simulink model "ThermalModel"  (R2021a)
settings: Solver=FixedStepAuto  StartTime=0.0  StopTime=860  FixedStep=0.1  RelTol=1e-3
values from neighbouring files (symbols this model uses):
  ACderate = 0.7910    (= 0.791)    [simvar.m]
  airtemp = 20    [simvar.m]
  CoreDm = 0.07    [simvar.m]
  CoreRm = 0.250/2    (= 0.125)    [simvar.m]
  Di = 0.085    [Optomised_simvar.m]    (also in simvar.m)
  Dm = 0.08    [simvar.m]
  Hi = 0.250    (= 0.25)    [Optomised_simvar.m]    (also in simvar.m)
  La = 1    [Optomised_simvar.m]    (also in simvar.m = 1.5)
  Li = 0.488    [Optomised_simvar.m]    (also in simvar.m)
  Lw = 1    [Optomised_simvar.m]    (also in simvar.m = 1.5)
  Nl = 20    [simvar.m]
  Nt = 7    [simvar.m]
  Nv = 14    [simvar.m]
  PDi = 0.03    [Optomised_simvar.m]    (also in simvar.m = 0.01)
  PDm = 0.01    [simvar.m]
  PLi = 1    [Optomised_simvar.m]    (also in simvar.m = 3.2)
  PLm = 0.721    [simvar.m]
  PSplit = 0.95    [simvar.m]
  Rm = 0.268/2    (= 0.134)    [simvar.m]
  StartTempI = 295    [simvar.m]
  StartTempM = 291    [simvar.m]
libraries: fl_lib x50, nesl_utility x20
settings Model: Creator=Henry  LastModifiedBy=Henry
settings SolverCC: AlgebraicLoopSolver=TrustRegion
settings DataIOCC: ReturnWorkspaceOutputs=off
settings DebuggingCC: SFMachineParentedDataDiag=warning  ArithmeticOperatorsInVariantConditions=warning
settings SFSimCC: SimUseLocalCustomCode=off  CustomCodeUndefinedFunction=UseInterfaceOnly
settings RTWCC: RTWUseLocalCustomCode=off

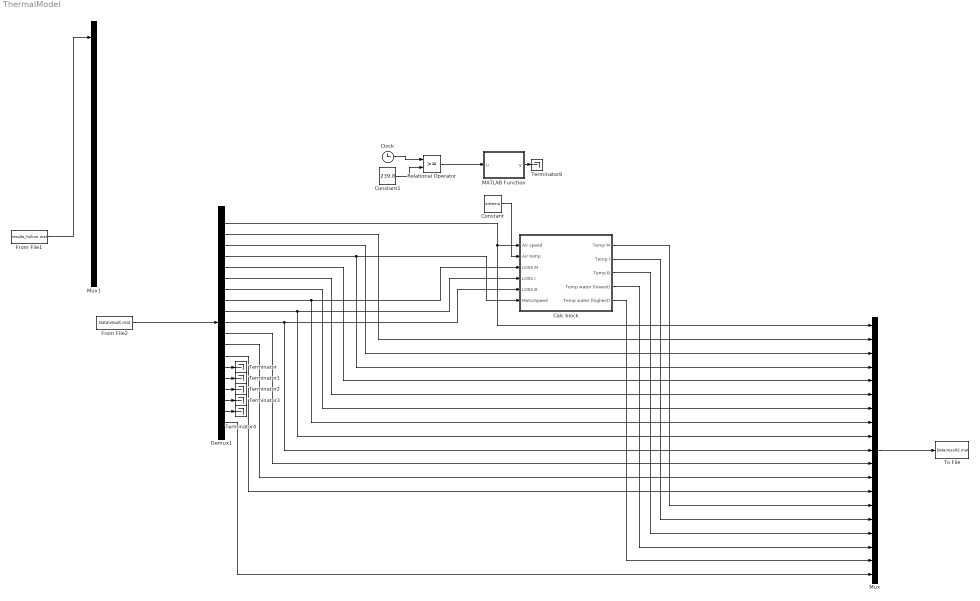
== system ThermalModel ==
  Calc block : Subsystem
  Clock : Clock
  Constant : Constant  Value=airtemp
  Constant1 : Constant  Value=239.8
  Demux1 : Demux  Outputs=19
  From File1 : FromFile  FileName=results_fullrun.mat  SampleTime=0
  From File2 : FromFile  FileName=Data\result.mat  SampleTime=0
  MATLAB Function : MATLAB Function  TreatAsAtomicUnit=on
  Mux : Mux  Inputs=19
  Mux1 : Mux  Inputs=8
  Relational Operator : RelationalOperator  OutDataTypeStr=boolean  RndMeth=Simplest
  Terminator{,1..4,8} (6 alike) : Terminator
  To File : ToFile  Filename=Data/result2.mat  MatrixName=Result  SaveFormat=Timeseries
  wires:
  Constant/1 -> Calc block/2(Air temp)
  Demux1/9 -> Calc block/4(LOSS I), Mux/9
  Demux1/8 -> Calc block/3(LOSS M), Mux/8
  Demux1/4 -> Calc block/6(MotorSpeed), Mux/4
  Demux1/10 -> Calc block/5(LOSS B), Mux/10
  Calc block/1(Temp M) -> Mux/14
  Calc block/2(Temp I) -> Mux/15
  Calc block/3(Temp B) -> Mux/16
  Calc block/4(Temp water (lowest)) -> Mux/17
  Calc block/5(Temp water (highest)) -> Mux/18
  Demux1/1 -> Mux/1, Calc block/1(Air speed)
  Clock/1 -> Relational Operator/1
  Constant1/1 -> Relational Operator/2
  Relational Operator/1 -> MATLAB Function/1(u)
  MATLAB Function/1(y) -> Terminator8/1
  Demux1/2 -> Mux/2
  Demux1/3 -> Mux/3
  Demux1/5 -> Mux/5
  Demux1/6 -> Mux/6
  Demux1/11 -> Mux/11
  Demux1/12 -> Mux/12
  Demux1/13 -> Mux/13
  Demux1/19 -> Mux/19
  Demux1/7 -> Mux/7
  Mux/1 -> To File/1
  Demux1/14 -> Terminator/1
  Demux1/15 -> Terminator1/1
  Demux1/16 -> Terminator2/1
  Demux1/17 -> Terminator3/1
  Demux1/18 -> Terminator4/1
  From File1/1 -> Mux1/1
  From File2/1 -> Demux1/1

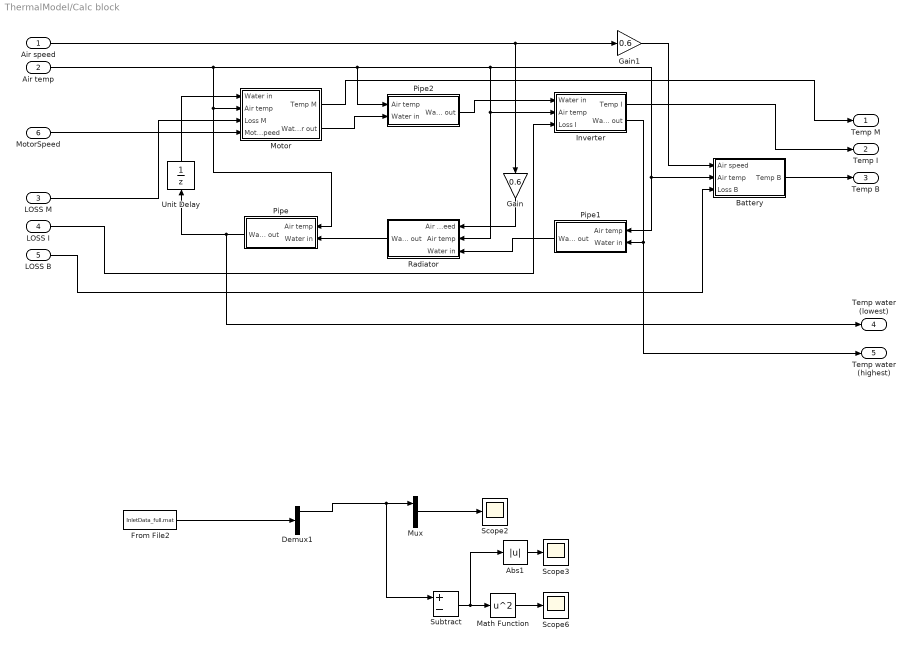
== system ThermalModel/Calc block ==
  Air speed : Inport
  Air temp : Inport  Port=2
  LOSS M : Inport  Port=3
  LOSS I : Inport  Port=4
  LOSS B : Inport  Port=5
  MotorSpeed : Inport  Port=6
  Abs1 : Abs
  Battery : Subsystem
  Demux1 : Demux  Outputs=3
  From File2 : FromFile  FileName=InletData_full.mat  SampleTime=0
  Gain : Gain  Gain=0.6
  Gain1 : Gain  Gain=0.6
  Inverter : Subsystem
  Math Function : Math  Operator=square  SaturateOnIntegerOverflow=on
  Motor : Subsystem
  Mux : Mux  Inputs=2
  Pipe : Subsystem
  Pipe1 : Subsystem
  Pipe2 : Subsystem
  Radiator : Subsystem
  Scope2 : Scope
  Scope3 : Scope
  Scope6 : Scope
  Subtract : Sum  Inputs=+-
  Unit Delay : UnitDelay  InitialCondition=20  SampleTime=-1  HasFrameUpgradeWarning=on
  Temp M : Outport  VectorParamsAs1DForOutWhenUnconnected=off
  Temp I : Outport  Port=2  VectorParamsAs1DForOutWhenUnconnected=off
  Temp B : Outport  Port=3  VectorParamsAs1DForOutWhenUnconnected=off
  Temp water (lowest) : Outport  Port=4  VectorParamsAs1DForOutWhenUnconnected=off
  Temp water (highest) : Outport  Port=5  VectorParamsAs1DForOutWhenUnconnected=off
  wires:
  Pipe/1(Water out) -> Unit Delay/1, Temp water (lowest)/1
  Battery/1(Temp B) -> Temp B/1
  Motor/1(Temp M) -> Temp M/1
  LOSS M/1 -> Motor/3(Loss M)
  Inverter/1(Temp I) -> Temp I/1
  LOSS B/1 -> Battery/3(Loss B)
  LOSS I/1 -> Inverter/3(Loss I)
  Air speed/1 -> Gain/1, Gain1/1
  Air temp/1 -> Pipe2/1(Air temp), Pipe1/1(Air temp), Battery/2(Air temp), Inverter/2(Air temp), Radiator/2(Air temp), Pipe/1(Air temp), Motor/2(Air temp)
  Pipe2/1(Water out) -> Inverter/1(Water in)
  Inverter/2(Water out) -> Pipe1/2(Water in), Temp water (highest)/1
  Motor/2(Water out) -> Pipe2/2(Water in)
  MotorSpeed/1 -> Motor/4(MotorSpeed)
  Unit Delay/1 -> Motor/1(Water in)
  Gain/1 -> Radiator/1(Air speed)
  Radiator/1(Water out) -> Pipe/2(Water in)
  Gain1/1 -> Battery/1(Air speed)
  Pipe1/1(Water out) -> Radiator/3(Water in)
  From File2/1 -> Demux1/1
  Demux1/1 -> Subtract/1, Mux/1
  Mux/1 -> Scope2/1
  Subtract/1 -> Abs1/1, Math Function/1
  Math Function/1 -> Scope6/1
  Abs1/1 -> Scope3/1

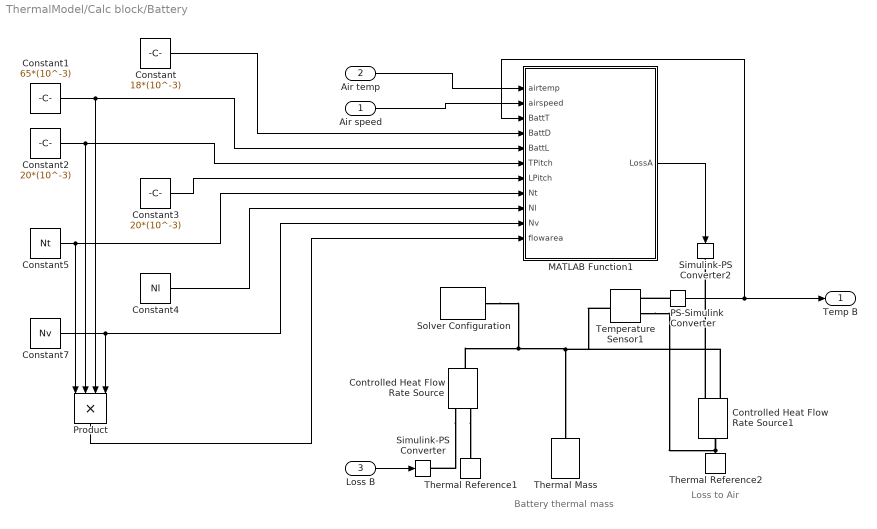
== system ThermalModel/Calc block/Battery ==
  note: Battery thermal mass
  note: Loss to Air
  Air speed : Inport
  Air temp : Inport  Port=2
  Loss B : Inport  Port=3
  Constant : Constant  Value=18*(10^-3)
  Constant1 : Constant  Value=65*(10^-3)
  Constant2 : Constant  Value=20*(10^-3)
  Constant3 : Constant  Value=20*(10^-3)
  Constant4 : Constant  Value=Nl
  Constant5 : Constant  Value=Nt
  Constant7 : Constant  Value=Nv
  Controlled Heat Flow Rate Source : fl_lib/Thermal/Thermal Sources/Controlled Heat Flow Rate Source
  Controlled Heat Flow Rate Source1 : fl_lib/Thermal/Thermal Sources/Controlled Heat Flow Rate Source
  MATLAB Function1 : MATLAB Function  TreatAsAtomicUnit=on
  PS-Simulink Converter : nesl_utility/PS-Simulink Converter  PhysicalDomain=network_engine_domain  SubClassName=ps_output  LeftPortType=input  RightPortType=output  PseudoPeriodic=off  Frequencies=[]  Unit=inherit  AffineConversion=off
      settings: SourceProductBaseCode=PW,SS
  Product : Product  Inputs=4
  Simulink-PS Converter : nesl_utility/Simulink-PS Converter  PhysicalDomain=network_engine_domain  SubClassName=ps_input  LeftPortType=input  RightPortType=output  PseudoPeriodic=off  Frequencies=[]  NoiseDistribution=none  NoiseParameters=[]  Unit=1  AffineConversion=off  FilteringAndDerivatives=provide  SimscapeFilterOrder=1  InputFilterTimeConstant=0.001  UdotUserProvided=0
      settings: SourceProductBaseCode=PW,SS
  Simulink-PS Converter2 : nesl_utility/Simulink-PS Converter  PhysicalDomain=network_engine_domain  SubClassName=ps_input  LeftPortType=input  RightPortType=output  PseudoPeriodic=off  Frequencies=[]  NoiseDistribution=none  NoiseParameters=[]  Unit=1  AffineConversion=off  FilteringAndDerivatives=provide  SimscapeFilterOrder=1  InputFilterTimeConstant=0.001  UdotUserProvided=0
      settings: SourceProductBaseCode=PW,SS
  Solver Configuration : nesl_utility/Solver Configuration  PhysicalDomain=network_engine_domain  SubClassName=solver  LeftPortType=input  RightPortType=generic  Tones=[]  Harmonics=[]  SimulateNoise=off  Profile=off  UseLocalSampling=off  EnableSwitchedLinearOptims=on  FrequencyDomain=off  UseCCode=off  RelTol=0.001  AbsTol=1e-06  MinStep=1e-09  ToWorkspace=off  RevertToSquareIcSolve=off  NumHomotopyIterations=100  PhasorMode=off  PhasorModeNumHarmonics=1  DoDC=off  ResidualTolerance=1e-09  UseLocalSolver=off  LocalSolverChoice=NE_BACKWARD_EULER_ADVANCER  LocalSolverSampleTime=0.001  DoFixedCost=off  MaxNonlinIter=3  MaxModeIter=2  ComputeImpulses=off  ImpulseIterations=2  LinearAlgebra=auto  EquationFormulation=NE_TIME_EF  DelaysMemoryBudget=2048  AutomaticFiltering=on  FilteringTimeConstant=0.001  PartitionStorageMethod=AS_NEEDED  PartitionMemoryBudget=1024  PartitionMethod=ROBUST
      settings: SourceProductBaseCode=PW,SS
  Temperature Sensor1 : fl_lib/Thermal/Thermal Sensors/Temperature Sensor
  Thermal Mass : fl_lib/Thermal/Thermal Elements/Thermal Mass  mass=Nt*Nl*Nv*0.045 kg  sp_heat=823 J/kg/K  T_specify=on  T_priority=High  T=300 K  T_nominal_specify=off  T_nominal_unit=K  T_nominal_value=1  Q_specify=off  Q_priority=None  Q=0 W  Q_nominal_specify=off  Q_nominal_unit=W  Q_nominal_value=1
  Thermal Reference1 : fl_lib/Thermal/Thermal Elements/Thermal Reference
  Thermal Reference2 : fl_lib/Thermal/Thermal Elements/Thermal Reference
  Temp B : Outport  VectorParamsAs1DForOutWhenUnconnected=off
  wires:
  Air temp/1 -> MATLAB Function1/1(airtemp)
  Air speed/1 -> MATLAB Function1/2(airspeed)
  Loss B/1 -> Simulink-PS Converter/1
  MATLAB Function1/1(LossA) -> Simulink-PS Converter2/1
  PS-Simulink Converter/1 -> Temp B/1, MATLAB Function1/3(BattT)
  Constant/1 -> MATLAB Function1/4(BattD)
  Constant1/1 -> MATLAB Function1/5(BattL), Product/3
  Constant2/1 -> MATLAB Function1/6(TPitch), Product/2
  Constant3/1 -> MATLAB Function1/7(LPitch)
  Constant5/1 -> MATLAB Function1/8(Nt), Product/1
  Constant4/1 -> MATLAB Function1/9(Nl)
  Product/1 -> MATLAB Function1/11(flowarea)
  Constant7/1 -> MATLAB Function1/10(Nv), Product/4
  connections:
  Controlled Heat Flow Rate Source/LConn1 -- Solver Configuration/RConn1 -- Temperature Sensor1/LConn1 -- Controlled Heat Flow Rate Source1/RConn2 -- Thermal Mass/LConn1
  Controlled Heat Flow Rate Source/RConn2 -- Thermal Reference1/LConn1
  Controlled Heat Flow Rate Source/RConn1 -- Simulink-PS Converter/RConn1
  Controlled Heat Flow Rate Source1/RConn1 -- Simulink-PS Converter2/RConn1
  Thermal Reference2/LConn1 -- Temperature Sensor1/RConn1 -- Controlled Heat Flow Rate Source1/LConn1
  PS-Simulink Converter/LConn1 -- Temperature Sensor1/RConn2

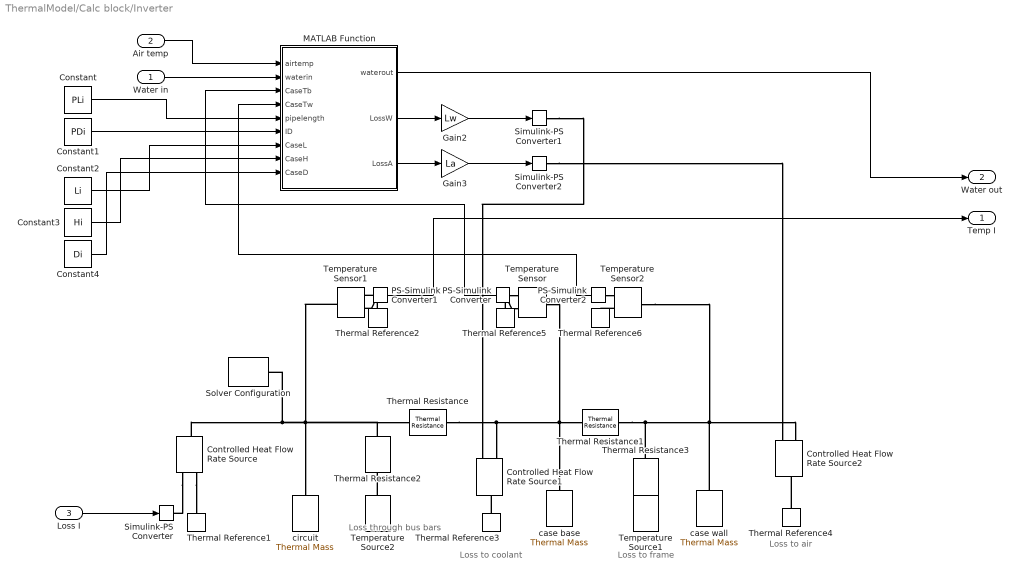
== system ThermalModel/Calc block/Inverter ==
  note: Loss to coolant
  note: Loss to air
  note: Loss through
      | bus bars
  note: Loss to frame
  Water in : Inport
  Air temp : Inport  Port=2
  Loss I : Inport  Port=3
  " case base" : fl_lib/Thermal/Thermal Elements/Thermal Mass  mass=MIbf kg  sp_heat=CpIb J/kg/K  T_specify=on  T_priority=High  T=StartTempI K  T_nominal_specify=off  T_nominal_unit=K  T_nominal_value=1  Q_specify=off  Q_priority=None  Q=0 W  Q_nominal_specify=off  Q_nominal_unit=W  Q_nominal_value=1
  " case wall" : fl_lib/Thermal/Thermal Elements/Thermal Mass  mass=MIbw kg  sp_heat=CpIb J/kg/K  T_specify=on  T_priority=High  T=StartTempI K  T_nominal_specify=off  T_nominal_unit=K  T_nominal_value=1  Q_specify=off  Q_priority=None  Q=0 W  Q_nominal_specify=off  Q_nominal_unit=W  Q_nominal_value=1
  Constant : Constant  Value=PLi
  Constant1 : Constant  Value=PDi
  Constant2 : Constant  Value=Li
  Constant3 : Constant  Value=Hi
  Constant4 : Constant  Value=Di
  Controlled Heat Flow Rate Source : fl_lib/Thermal/Thermal Sources/Controlled Heat Flow Rate Source
  Controlled Heat Flow Rate Source1 : fl_lib/Thermal/Thermal Sources/Controlled Heat Flow Rate Source
  Controlled Heat Flow Rate Source2 : fl_lib/Thermal/Thermal Sources/Controlled Heat Flow Rate Source
  Gain2 : Gain  Gain=Lw
  Gain3 : Gain  Gain=La
  MATLAB Function : MATLAB Function  TreatAsAtomicUnit=on
  PS-Simulink Converter : nesl_utility/PS-Simulink Converter  PhysicalDomain=network_engine_domain  SubClassName=ps_output  LeftPortType=input  RightPortType=output  PseudoPeriodic=off  Frequencies=[]  Unit=inherit  AffineConversion=off
      settings: SourceProductBaseCode=PW,SS
  PS-Simulink Converter1 : nesl_utility/PS-Simulink Converter  PhysicalDomain=network_engine_domain  SubClassName=ps_output  LeftPortType=input  RightPortType=output  PseudoPeriodic=off  Frequencies=[]  Unit=inherit  AffineConversion=off
      settings: SourceProductBaseCode=PW,SS
  PS-Simulink Converter2 : nesl_utility/PS-Simulink Converter  PhysicalDomain=network_engine_domain  SubClassName=ps_output  LeftPortType=input  RightPortType=output  PseudoPeriodic=off  Frequencies=[]  Unit=inherit  AffineConversion=off
      settings: SourceProductBaseCode=PW,SS
  Simulink-PS Converter : nesl_utility/Simulink-PS Converter  PhysicalDomain=network_engine_domain  SubClassName=ps_input  LeftPortType=input  RightPortType=output  PseudoPeriodic=off  Frequencies=[]  NoiseDistribution=none  NoiseParameters=[]  Unit=1  AffineConversion=off  FilteringAndDerivatives=provide  SimscapeFilterOrder=1  InputFilterTimeConstant=0.001  UdotUserProvided=0
      settings: SourceProductBaseCode=PW,SS
  Simulink-PS Converter1 : nesl_utility/Simulink-PS Converter  PhysicalDomain=network_engine_domain  SubClassName=ps_input  LeftPortType=input  RightPortType=output  PseudoPeriodic=off  Frequencies=[]  NoiseDistribution=none  NoiseParameters=[]  Unit=1  AffineConversion=off  FilteringAndDerivatives=provide  SimscapeFilterOrder=1  InputFilterTimeConstant=0.001  UdotUserProvided=0
      settings: SourceProductBaseCode=PW,SS
  Simulink-PS Converter2 : nesl_utility/Simulink-PS Converter  PhysicalDomain=network_engine_domain  SubClassName=ps_input  LeftPortType=input  RightPortType=output  PseudoPeriodic=off  Frequencies=[]  NoiseDistribution=none  NoiseParameters=[]  Unit=1  AffineConversion=off  FilteringAndDerivatives=provide  SimscapeFilterOrder=1  InputFilterTimeConstant=0.001  UdotUserProvided=0
      settings: SourceProductBaseCode=PW,SS
  Solver Configuration : nesl_utility/Solver Configuration  PhysicalDomain=network_engine_domain  SubClassName=solver  LeftPortType=input  RightPortType=generic  Tones=[]  Harmonics=[]  SimulateNoise=off  Profile=off  UseLocalSampling=off  EnableSwitchedLinearOptims=on  FrequencyDomain=off  UseCCode=off  RelTol=0.001  AbsTol=1e-06  MinStep=1e-09  ToWorkspace=off  RevertToSquareIcSolve=off  NumHomotopyIterations=100  PhasorMode=off  PhasorModeNumHarmonics=1  DoDC=off  ResidualTolerance=1e-09  UseLocalSolver=off  LocalSolverChoice=NE_BACKWARD_EULER_ADVANCER  LocalSolverSampleTime=0.001  DoFixedCost=off  MaxNonlinIter=3  MaxModeIter=2  ComputeImpulses=off  ImpulseIterations=2  LinearAlgebra=auto  EquationFormulation=NE_TIME_EF  DelaysMemoryBudget=2048  AutomaticFiltering=on  FilteringTimeConstant=0.001  PartitionStorageMethod=AS_NEEDED  PartitionMemoryBudget=1024  PartitionMethod=ROBUST
      settings: SourceProductBaseCode=PW,SS
  Temperature Sensor : fl_lib/Thermal/Thermal Sensors/Temperature Sensor
  Temperature Sensor1 : fl_lib/Thermal/Thermal Sensors/Temperature Sensor
  Temperature Sensor2 : fl_lib/Thermal/Thermal Sensors/Temperature Sensor
  Temperature Source1 : fl_lib/Thermal/Thermal Sources/Temperature Source  temperature=293.15 K
  Temperature Source2 : fl_lib/Thermal/Thermal Sources/Temperature Source  temperature=293.15 K
  Thermal Reference{1..6} (6 alike) : fl_lib/Thermal/Thermal Elements/Thermal Reference
  Thermal Resistance : fl_lib/Thermal/Thermal Elements/Thermal Resistance  resistance=Rcb K/W  T_specify=off  T_priority=None  T=0 K  T_nominal_specify=off  T_nominal_unit=K  T_nominal_value=1  Q_specify=off  Q_priority=None  Q=0 W  Q_nominal_specify=off  Q_nominal_unit=W  Q_nominal_value=1
      settings: SourceProductBaseCode=SS
  Thermal Resistance1 : fl_lib/Thermal/Thermal Elements/Thermal Resistance  resistance=Rba K/W  T_specify=off  T_priority=None  T=0 K  T_nominal_specify=off  T_nominal_unit=K  T_nominal_value=1  Q_specify=off  Q_priority=None  Q=0 W  Q_nominal_specify=off  Q_nominal_unit=W  Q_nominal_value=1
      settings: SourceProductBaseCode=SS
  Thermal Resistance2 : fl_lib/Thermal/Thermal Elements/Thermal Resistance  resistance=Rcbb K/W  T_specify=off  T_priority=None  T=0 K  T_nominal_specify=off  T_nominal_unit=K  T_nominal_value=1  Q_specify=off  Q_priority=None  Q=0 W  Q_nominal_specify=off  Q_nominal_unit=W  Q_nominal_value=1
      settings: SourceProductBaseCode=SS
  Thermal Resistance3 : fl_lib/Thermal/Thermal Elements/Thermal Resistance  resistance=Rcf K/W  T_specify=off  T_priority=None  T=0 K  T_nominal_specify=off  T_nominal_unit=K  T_nominal_value=1  Q_specify=off  Q_priority=None  Q=0 W  Q_nominal_specify=off  Q_nominal_unit=W  Q_nominal_value=1
      settings: SourceProductBaseCode=SS
  circuit : fl_lib/Thermal/Thermal Elements/Thermal Mass  mass=MIc kg  sp_heat=CpIc J/kg/K  T_specify=on  T_priority=High  T=StartTempI K  T_nominal_specify=off  T_nominal_unit=K  T_nominal_value=1  Q_specify=off  Q_priority=None  Q=0 W  Q_nominal_specify=off  Q_nominal_unit=W  Q_nominal_value=1
  Temp I : Outport  VectorParamsAs1DForOutWhenUnconnected=off
  Water out : Outport  Port=2  VectorParamsAs1DForOutWhenUnconnected=off
  wires:
  PS-Simulink Converter1/1 -> Temp I/1
  Air temp/1 -> MATLAB Function/1(airtemp)
  Water in/1 -> MATLAB Function/2(waterin)
  MATLAB Function/1(waterout) -> Water out/1
  PS-Simulink Converter/1 -> MATLAB Function/3(CaseTb)
  MATLAB Function/2(LossW) -> Gain2/1
  MATLAB Function/3(LossA) -> Gain3/1
  Constant/1 -> MATLAB Function/5(pipelength)
  Constant1/1 -> MATLAB Function/6(ID)
  Constant2/1 -> MATLAB Function/7(CaseL)
  Constant3/1 -> MATLAB Function/8(CaseH)
  Constant4/1 -> MATLAB Function/9(CaseD)
  PS-Simulink Converter2/1 -> MATLAB Function/4(CaseTw)
  Loss I/1 -> Simulink-PS Converter/1
  Gain2/1 -> Simulink-PS Converter1/1
  Gain3/1 -> Simulink-PS Converter2/1
  connections:
  Thermal Reference3/LConn1 -- Controlled Heat Flow Rate Source1/LConn1
  Thermal Resistance/RConn1 -- Temperature Sensor/LConn1 -- Thermal Resistance1/LConn1 -- " case base"/LConn1 -- Controlled Heat Flow Rate Source1/RConn2
  PS-Simulink Converter/LConn1 -- Temperature Sensor/RConn2
  Controlled Heat Flow Rate Source/RConn2 -- Thermal Reference1/LConn1
  Controlled Heat Flow Rate Source/RConn1 -- Simulink-PS Converter/RConn1
  Thermal Resistance1/RConn1 -- Thermal Resistance3/LConn1 -- Temperature Sensor2/LConn1 -- " case wall"/LConn1 -- Controlled Heat Flow Rate Source2/RConn2
  PS-Simulink Converter1/LConn1 -- Temperature Sensor1/RConn2
  Simulink-PS Converter1/RConn1 -- Controlled Heat Flow Rate Source1/RConn1
  Simulink-PS Converter2/RConn1 -- Controlled Heat Flow Rate Source2/RConn1
  Thermal Reference4/LConn1 -- Controlled Heat Flow Rate Source2/LConn1
  Thermal Reference2/LConn1 -- Temperature Sensor1/RConn1
  Thermal Reference5/LConn1 -- Temperature Sensor/RConn1
  Controlled Heat Flow Rate Source/LConn1 -- Thermal Resistance2/LConn1 -- Thermal Resistance/LConn1 -- Temperature Sensor1/LConn1 -- circuit/LConn1 -- Solver Configuration/RConn1
  PS-Simulink Converter2/LConn1 -- Temperature Sensor2/RConn2
  Temperature Sensor2/RConn1 -- Thermal Reference6/LConn1
  Temperature Source1/LConn1 -- Thermal Resistance3/RConn1
  Temperature Source2/LConn1 -- Thermal Resistance2/RConn1

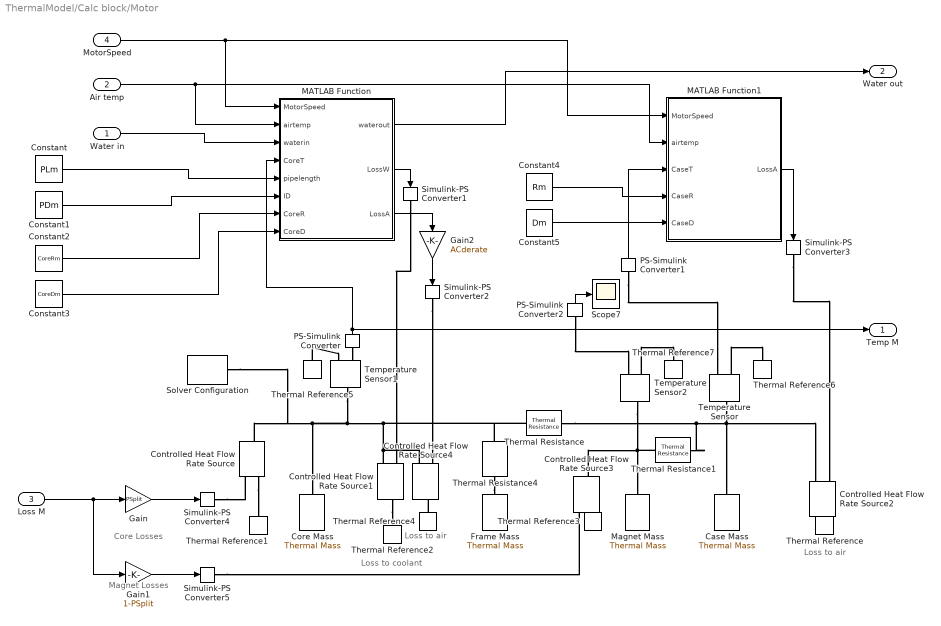
== system ThermalModel/Calc block/Motor ==
  note: Core Losses
  note: Loss to air
  note: Loss to coolant
  note: Loss to air
  note: Magnet Losses
  Water in : Inport
  Air temp : Inport  Port=2
  Loss M : Inport  Port=3
  MotorSpeed : Inport  Port=4
  " Case Mass" : fl_lib/Thermal/Thermal Elements/Thermal Mass  mass=Mcase kg  sp_heat=Cpcase J/kg/K  T_specify=on  T_priority=High  T=StartTempM K  T_nominal_specify=off  T_nominal_unit=K  T_nominal_value=1  Q_specify=off  Q_priority=None  Q=0 W  Q_nominal_specify=off  Q_nominal_unit=W  Q_nominal_value=1
  " Frame Mass" : fl_lib/Thermal/Thermal Elements/Thermal Mass  mass=30 kg  sp_heat=447 J/kg/K  T_specify=on  T_priority=High  T=StartTempM K  T_nominal_specify=off  T_nominal_unit=K  T_nominal_value=1  Q_specify=off  Q_priority=None  Q=0 W  Q_nominal_specify=off  Q_nominal_unit=W  Q_nominal_value=1
  " Magnet Mass" : fl_lib/Thermal/Thermal Elements/Thermal Mass  mass=Mmag kg  sp_heat=Cpmag J/kg/K  T_specify=on  T_priority=High  T=StartTempM K  T_nominal_specify=off  T_nominal_unit=K  T_nominal_value=1  Q_specify=off  Q_priority=None  Q=0 W  Q_nominal_specify=off  Q_nominal_unit=W  Q_nominal_value=1
  Constant : Constant  Value=PLm
  Constant1 : Constant  Value=PDm
  Constant2 : Constant  Value=CoreRm
  Constant3 : Constant  Value=CoreDm
  Constant4 : Constant  Value=Rm
  Constant5 : Constant  Value=Dm
  Controlled Heat Flow Rate Source{,1..4} (5 alike) : fl_lib/Thermal/Thermal Sources/Controlled Heat Flow Rate Source
  Core Mass : fl_lib/Thermal/Thermal Elements/Thermal Mass  mass=Mc kg  sp_heat=Cpcore J/kg/K  T_specify=on  T_priority=High  T=StartTempM K  T_nominal_specify=off  T_nominal_unit=K  T_nominal_value=1  Q_specify=off  Q_priority=None  Q=0 W  Q_nominal_specify=off  Q_nominal_unit=W  Q_nominal_value=1
  Gain : Gain  Gain=PSplit
  Gain1 : Gain  Gain=1-PSplit
  Gain2 : Gain  Gain=ACderate
  MATLAB Function : MATLAB Function  TreatAsAtomicUnit=on
  MATLAB Function1 : MATLAB Function  TreatAsAtomicUnit=on
  PS-Simulink Converter : nesl_utility/PS-Simulink Converter  PhysicalDomain=network_engine_domain  SubClassName=ps_output  LeftPortType=input  RightPortType=output  PseudoPeriodic=off  Frequencies=[]  Unit=inherit  AffineConversion=off
      settings: SourceProductBaseCode=PW,SS
  PS-Simulink Converter1 : nesl_utility/PS-Simulink Converter  PhysicalDomain=network_engine_domain  SubClassName=ps_output  LeftPortType=input  RightPortType=output  PseudoPeriodic=off  Frequencies=[]  Unit=inherit  AffineConversion=off
      settings: SourceProductBaseCode=PW,SS
  PS-Simulink Converter2 : nesl_utility/PS-Simulink Converter  PhysicalDomain=network_engine_domain  SubClassName=ps_output  LeftPortType=input  RightPortType=output  PseudoPeriodic=off  Frequencies=[]  Unit=inherit  AffineConversion=off
      settings: SourceProductBaseCode=PW,SS
  Scope7 : Scope
  Simulink-PS Converter{1..5} (5 alike) : nesl_utility/Simulink-PS Converter  PhysicalDomain=network_engine_domain  SubClassName=ps_input  LeftPortType=input  RightPortType=output  PseudoPeriodic=off  Frequencies=[]  NoiseDistribution=none  NoiseParameters=[]  Unit=1  AffineConversion=off  FilteringAndDerivatives=provide  SimscapeFilterOrder=1  InputFilterTimeConstant=0.001  UdotUserProvided=0
      settings: SourceProductBaseCode=PW,SS
  Solver Configuration : nesl_utility/Solver Configuration  PhysicalDomain=network_engine_domain  SubClassName=solver  LeftPortType=input  RightPortType=generic  Tones=[]  Harmonics=[]  SimulateNoise=off  Profile=off  UseLocalSampling=off  EnableSwitchedLinearOptims=on  FrequencyDomain=off  UseCCode=off  RelTol=0.001  AbsTol=1e-06  MinStep=1e-09  ToWorkspace=off  RevertToSquareIcSolve=off  NumHomotopyIterations=100  PhasorMode=off  PhasorModeNumHarmonics=1  DoDC=off  ResidualTolerance=1e-09  UseLocalSolver=off  LocalSolverChoice=NE_BACKWARD_EULER_ADVANCER  LocalSolverSampleTime=0.001  DoFixedCost=off  MaxNonlinIter=3  MaxModeIter=2  ComputeImpulses=off  ImpulseIterations=2  LinearAlgebra=auto  EquationFormulation=NE_TIME_EF  DelaysMemoryBudget=2048  AutomaticFiltering=on  FilteringTimeConstant=0.001  PartitionStorageMethod=AS_NEEDED  PartitionMemoryBudget=1024  PartitionMethod=ROBUST
      settings: SourceProductBaseCode=PW,SS
  Temperature Sensor : fl_lib/Thermal/Thermal Sensors/Temperature Sensor
  Temperature Sensor1 : fl_lib/Thermal/Thermal Sensors/Temperature Sensor
  Temperature Sensor2 : fl_lib/Thermal/Thermal Sensors/Temperature Sensor
  Thermal Reference{,1..7} (8 alike) : fl_lib/Thermal/Thermal Elements/Thermal Reference
  Thermal Resistance : fl_lib/Thermal/Thermal Elements/Thermal Resistance  resistance=Rcc K/W  T_specify=off  T_priority=None  T=0 K  T_nominal_specify=off  T_nominal_unit=K  T_nominal_value=1  Q_specify=off  Q_priority=None  Q=0 W  Q_nominal_specify=off  Q_nominal_unit=W  Q_nominal_value=1
      settings: SourceProductBaseCode=SS
  Thermal Resistance1 : fl_lib/Thermal/Thermal Elements/Thermal Resistance  resistance=Rmc K/W  T_specify=off  T_priority=None  T=0 K  T_nominal_specify=off  T_nominal_unit=K  T_nominal_value=1  Q_specify=off  Q_priority=None  Q=0 W  Q_nominal_specify=off  Q_nominal_unit=W  Q_nominal_value=1
      settings: SourceProductBaseCode=SS
  Thermal Resistance4 : fl_lib/Thermal/Thermal Elements/Thermal Resistance  resistance=Rcf K/W  T_specify=off  T_priority=None  T=0 K  T_nominal_specify=off  T_nominal_unit=K  T_nominal_value=1  Q_specify=off  Q_priority=None  Q=0 W  Q_nominal_specify=off  Q_nominal_unit=W  Q_nominal_value=1
      settings: SourceProductBaseCode=SS
  Temp M : Outport  VectorParamsAs1DForOutWhenUnconnected=off
  Water out : Outport  Port=2  VectorParamsAs1DForOutWhenUnconnected=off
  wires:
  PS-Simulink Converter/1 -> Temp M/1, MATLAB Function/4(CoreT)
  Air temp/1 -> MATLAB Function1/2(airtemp), MATLAB Function/2(airtemp)
  Water in/1 -> MATLAB Function/3(waterin)
  MATLAB Function/2(LossW) -> Simulink-PS Converter1/1
  MATLAB Function/3(LossA) -> Gain2/1
  MATLAB Function/1(waterout) -> Water out/1
  MATLAB Function1/1(LossA) -> Simulink-PS Converter3/1
  PS-Simulink Converter1/1 -> MATLAB Function1/3(CaseT)
  Loss M/1 -> Gain/1, Gain1/1
  Gain/1 -> Simulink-PS Converter4/1
  Gain1/1 -> Simulink-PS Converter5/1
  Constant/1 -> MATLAB Function/5(pipelength)
  Constant1/1 -> MATLAB Function/6(ID)
  Constant2/1 -> MATLAB Function/7(CoreR)
  Constant3/1 -> MATLAB Function/8(CoreD)
  Constant4/1 -> MATLAB Function1/4(CaseR)
  Constant5/1 -> MATLAB Function1/5(CaseD)
  MotorSpeed/1 -> MATLAB Function/1(MotorSpeed), MATLAB Function1/1(MotorSpeed)
  PS-Simulink Converter2/1 -> Scope7/1
  Gain2/1 -> Simulink-PS Converter2/1
  connections:
  Thermal Resistance/RConn1 -- Thermal Resistance1/RConn1 -- Temperature Sensor/LConn1 -- " Case Mass"/LConn1 -- Controlled Heat Flow Rate Source2/RConn2
  Simulink-PS Converter4/RConn1 -- Controlled Heat Flow Rate Source/RConn1
  Thermal Reference/LConn1 -- Controlled Heat Flow Rate Source2/LConn1
  Controlled Heat Flow Rate Source/RConn2 -- Thermal Reference1/LConn1
  PS-Simulink Converter/LConn1 -- Temperature Sensor1/RConn2
  Controlled Heat Flow Rate Source1/LConn1 -- Thermal Reference2/LConn1
  Thermal Reference3/LConn1 -- Controlled Heat Flow Rate Source3/RConn2
  Thermal Reference4/LConn1 -- Controlled Heat Flow Rate Source4/LConn1
  Simulink-PS Converter1/RConn1 -- Controlled Heat Flow Rate Source1/RConn1
  Simulink-PS Converter2/RConn1 -- Controlled Heat Flow Rate Source4/RConn1
  Simulink-PS Converter3/RConn1 -- Controlled Heat Flow Rate Source2/RConn1
  PS-Simulink Converter1/LConn1 -- Temperature Sensor/RConn2
  Simulink-PS Converter5/RConn1 -- Controlled Heat Flow Rate Source3/RConn1
  Controlled Heat Flow Rate Source4/RConn2 -- Controlled Heat Flow Rate Source1/RConn2 -- Solver Configuration/RConn1 -- Controlled Heat Flow Rate Source/LConn1 -- Core Mass/LConn1 -- Temperature Sensor1/LConn1 -- Thermal Resistance/LConn1 -- Thermal Resistance4/LConn1
  Thermal Resistance4/RConn1 -- " Frame Mass"/LConn1
  Thermal Reference5/LConn1 -- Temperature Sensor1/RConn1
  Temperature Sensor/RConn1 -- Thermal Reference6/LConn1
  Controlled Heat Flow Rate Source3/LConn1 -- Temperature Sensor2/LConn1 -- Thermal Resistance1/LConn1 -- " Magnet Mass"/LConn1
  Temperature Sensor2/RConn1 -- Thermal Reference7/LConn1
  PS-Simulink Converter2/LConn1 -- Temperature Sensor2/RConn2

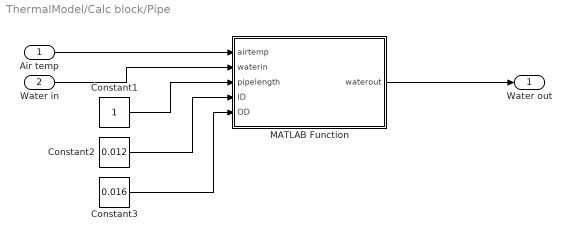
== system ThermalModel/Calc block/Pipe ==
  Air temp : Inport
  Water in : Inport  Port=2
  Constant1 : Constant
  Constant2 : Constant  Value=0.012
  Constant3 : Constant  Value=0.016
  MATLAB Function : MATLAB Function  TreatAsAtomicUnit=on
  Water out : Outport  VectorParamsAs1DForOutWhenUnconnected=off
  wires:
  MATLAB Function/1(waterout) -> Water out/1
  Constant1/1 -> MATLAB Function/3(pipelength)
  Water in/1 -> MATLAB Function/2(waterin)
  Air temp/1 -> MATLAB Function/1(airtemp)
  Constant2/1 -> MATLAB Function/4(ID)
  Constant3/1 -> MATLAB Function/5(OD)

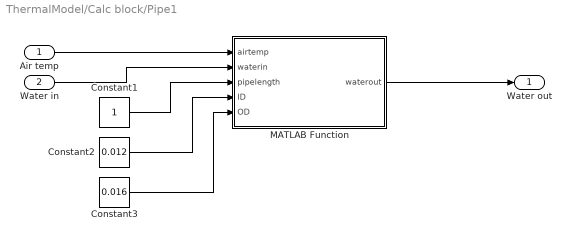
== system ThermalModel/Calc block/Pipe1 ==
  Air temp : Inport
  Water in : Inport  Port=2
  Constant1 : Constant
  Constant2 : Constant  Value=0.012
  Constant3 : Constant  Value=0.016
  MATLAB Function : MATLAB Function  TreatAsAtomicUnit=on
  Water out : Outport  VectorParamsAs1DForOutWhenUnconnected=off
  wires:
  MATLAB Function/1(waterout) -> Water out/1
  Constant1/1 -> MATLAB Function/3(pipelength)
  Water in/1 -> MATLAB Function/2(waterin)
  Air temp/1 -> MATLAB Function/1(airtemp)
  Constant2/1 -> MATLAB Function/4(ID)
  Constant3/1 -> MATLAB Function/5(OD)

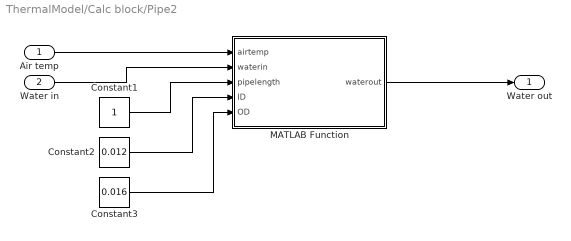
== system ThermalModel/Calc block/Pipe2 ==
  Air temp : Inport
  Water in : Inport  Port=2
  Constant1 : Constant
  Constant2 : Constant  Value=0.012
  Constant3 : Constant  Value=0.016
  MATLAB Function : MATLAB Function  TreatAsAtomicUnit=on
  Water out : Outport  VectorParamsAs1DForOutWhenUnconnected=off
  wires:
  MATLAB Function/1(waterout) -> Water out/1
  Constant1/1 -> MATLAB Function/3(pipelength)
  Water in/1 -> MATLAB Function/2(waterin)
  Air temp/1 -> MATLAB Function/1(airtemp)
  Constant2/1 -> MATLAB Function/4(ID)
  Constant3/1 -> MATLAB Function/5(OD)

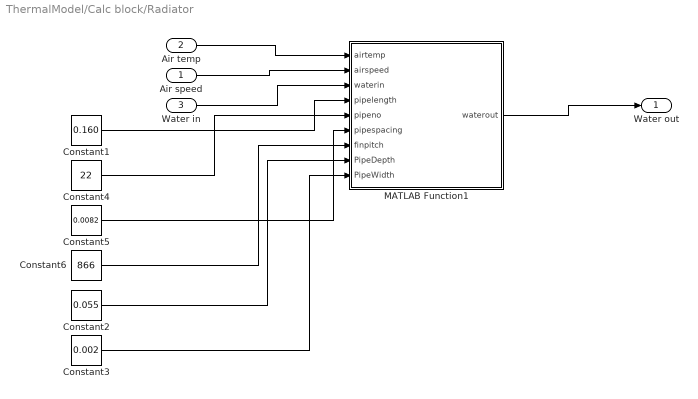
== system ThermalModel/Calc block/Radiator ==
  Air speed : Inport
  Air temp : Inport  Port=2
  Water in : Inport  Port=3
  Constant1 : Constant  Value=0.160
  Constant2 : Constant  Value=0.055
  Constant3 : Constant  Value=0.002
  Constant4 : Constant  Value=22
  Constant5 : Constant  Value=0.0082
  Constant6 : Constant  Value=866
  MATLAB Function1 : MATLAB Function  TreatAsAtomicUnit=on
  Water out : Outport  VectorParamsAs1DForOutWhenUnconnected=off
  wires:
  Air speed/1 -> MATLAB Function1/2(airspeed)
  Air temp/1 -> MATLAB Function1/1(airtemp)
  Water in/1 -> MATLAB Function1/3(waterin)
  MATLAB Function1/1(waterout) -> Water out/1
  Constant1/1 -> MATLAB Function1/4(pipelength)
  Constant2/1 -> MATLAB Function1/8(PipeDepth)
  Constant3/1 -> MATLAB Function1/9(PipeWidth)
  Constant4/1 -> MATLAB Function1/5(pipeno)
  Constant6/1 -> MATLAB Function1/7(finpitch)
  Constant5/1 -> MATLAB Function1/6(pipespacing)

== matlab function ThermalModel/Calc block/Motor/MATLAB Function ==
  data: MotorSpeed input; airtemp input; waterin input; CoreT input; waterout output; pipelength input; ID input; CoreR input; CoreD input; LossW output; LossA output
function [waterout,LossW,LossA] = MotCorefcn(MotorSpeed,airtemp,waterin,CoreT,pipelength,ID,CoreR,CoreD)

SurfSpeed = (abs(MotorSpeed)/CoreR);
CoreT = CoreT - 273.15;
L = pipelength;
AveWtemp = waterin;
dmw = 0.1;
u = (dmw/1000)/(pi()*((ID/2)^2));
filmT1 = (waterin + CoreT)/2;
filmT2 = (CoreT + airtemp)/2;

[Rew,Prw,Grw,kw,Cpw] = Variablefinder('water',filmT1,AveWtemp,u,ID);
[Rea,Pra,Gra,ka,Cpa] = Variablefinder('air',filmT2,airtemp,SurfSpeed,pi()*CoreR*2);

if Rew <= 2300
    Nuw = 3.66;     %value for laminar flow in a pipe with constant surface temp
elseif Rew<= 10000
    f = (0.79*log(Rew-1.64) )^(-2);
    Nuw = (f/8*(Rew-1000)*Prw)/(1+(12.7*((f/8)^(1/2))*(Prw^(2/3)-1)) );
else
    Nuw = 0.023*(Rew^(4/5))*(Prw^0.3);   %equation for turbulent flow in a cooling pipe
end

% Raa = Pra*Gra;  %calculate the rayleigh number
% Nua = (0.825 + ( (0.387*(Raa^(1/6))) / ((1 + ((0.492/Pra)^(9/16)))^(8/27)) ) )^2;
if Rea <= (5*10^5)
    Nua = 0.664*(Rea^(1/2))*(Pra^(1/3));
else
    Nua = ((0.037*(Rea^(4/5)))-871)*(Pra^(1/3));
end

h1 = Nuw*kw/(ID);
h2 = Nua*ka/pi()*CoreR*2;

R1 = 1/(pi()*(ID)*L*h1);

R2 = 1/((pi()*(CoreD)*2*CoreR*h2));

waterout = CoreT - (CoreT-waterin)*exp(-1/(dmw*Cpw*R1));

LossW = dmw*Cpw*(waterout - waterin);

LossA = (CoreT-airtemp)/R2;

end

== matlab function ThermalModel/Calc block/Motor/MATLAB Function1 ==
  data: MotorSpeed input; airtemp input; CaseT input; CaseR input; CaseD input; LossA output
function LossA  = MotCasefcn(MotorSpeed,airtemp,CaseT,CaseR,CaseD)

SurfSpeed = abs(MotorSpeed)/CaseR;
CaseT = CaseT - 273.15;
filmT1 = (CaseT + airtemp)/2;

[Rea,Pra,Gra,ka,Cpa] = Variablefinder('air',filmT1,airtemp,SurfSpeed,pi()*CaseR*2);

if Rea <= (5*10^5)
    Nua = 0.664*(Rea^(1/2))*(Pra^(1/3));
else
    Nua = ((0.037*(Rea^(4/5)))-871)*(Pra^(1/3));
end

h1 = Nua*ka/(2*CaseR*pi());

R1 = 1/((2*CaseR*pi())*CaseD*h1);

LossA = (CaseT-airtemp)/R1;

end

== matlab function ThermalModel/Calc block/Pipe1/MATLAB Function ==
  data: airtemp input; waterin input; waterout output; pipelength input; ID input; OD input
function waterout = Pipefcn(airtemp,waterin,pipelength,ID,OD)

L = pipelength;
AveWtemp = waterin;
kpipe = 0.13;
dm = 0.1;
u = (dm/1000)/(pi()*((ID/2)^2));
filmT1 = (waterin + airtemp)/2;
filmT2 = (waterin + airtemp)/2;

for x = 1:3
    [Rew,Prw,Grw,kw,Cpw] = Variablefinder('water',filmT1,AveWtemp,u,ID);
    [Rea,Pra,Gra,ka,Cpa] = Variablefinder('air',filmT2,airtemp,0,OD);
    
    if Rew <= 2300
        Nuw = 3.66;     %value for laminar flow in a pipe with constant surface temp
    else
       Nuw = 0.023*(Rew^(4/5))*(Prw^0.3);   %equation for turbulent flow in a cooling pipe
    end
    
    Raa = Pra*Gra;  %calculate the rayleigh number
    HorNua = (0.6 + ( (0.387*(Raa^(1/6))) / ((1 + ((0.559/Pra)^(9/16)))^(8/27)) ) )^2;
    VertNua = (0.825 + ( (0.387*(Raa^(1/6))) / ((1 + ((0.492/Pra)^(9/16)))^(8/27)) ) )^2;
    Nua = 1*HorNua + 0*VertNua;
    
    h1 = Nuw*kw/ID;
    h2 = Nua*ka/OD;

    R1 = 1/(2*pi()*(ID/2)*L*h1);
    R2 = (log((OD/2)/(ID/2)))/(2*pi()*L*kpipe);
    R3 = 1/(2*pi()*(OD/2)*L*h2);
    Rt = R1 + R2 + R3;
    
    waterout = airtemp - (airtemp-waterin)*exp(-1/(dm*Cpw*Rt));

    AveWtemp = (waterin + waterout)/2;
    AvedQ = dm*Cpw*(waterin - waterout);
    
    dTt = AveWtemp - airtemp;
    dT1 = dTt*(R1/Rt);
    dT3 = dTt*(R3/Rt);
    
    filmT1 = AveWtemp - (dT1/2);
    filmT2 = airtemp + (dT3/2);   
end

end

== matlab function ThermalModel/Calc block/Battery/MATLAB Function1 ==
  data: airtemp input; airspeed input; BattT input; BattD input; LossA output; BattL input; TPitch input; LPitch input; Nt input; Nl input; Nv input; flowarea input
function LossA  = Battfcn(airtemp,airspeed,BattT,BattD,BattL,TPitch,LPitch,Nt,Nl,Nv,flowarea)

BattT = BattT-273.15;

T = [250,275,300,325,350]-273.15;
mu = [1.599,1.725,1.846,1.962,2.075].*(10^-5);
rho = [1.412,1.284,1.177,1.086,1.009];

rho = interp1(T,rho,airtemp);
dm = flowarea*airspeed*rho;

 %Fmax = dm*airspeed;         %maximum force the air could exert on the battery air intake
 %Pmax = Fmax/flowarea;       %maximum guage pressure possible at air intake
Pmax = 0.5*rho*(airspeed^2);

mufs = interp1(T,mu,airtemp);
mus = interp1(T,mu,BattT);

filmT1 = (BattT + airtemp)/2;

[ReN,PrN,GrN,kN,CpaN] = Variablefinder('air',filmT1,airtemp,0,BattL*Nv);     %cells are verticaly oriented so the natural convection parameters are found using height not diameter

[Re,Pr,Gr,k,Cpa] = Variablefinder('air',filmT1,airtemp,airspeed,BattD);
for x = 1:5
    fric = (0.44 + (0.08*LPitch/BattD)/(((TPitch-BattD)/BattD)^(0.43+1.13*(BattD/LPitch))))*Re^(-0.15);     %friction coefficient for in-line pack
    Gmax = ( ((Pmax)*rho) / (2*fric*Nt*Nv*((mus/mufs)^0.14)) )^(1/2);          %maximum masss flow rate through battery based on max pressure at intake
    umax = (Gmax/(flowarea*rho))*(TPitch/(TPitch-BattD));                   %peak air speed within pack
    [Re,Pr,Gr,k,Cpa] = Variablefinder('air',filmT1,airtemp,umax,BattD);     %re-find variables based on speed
end

if Gmax > dm
    Gmax = dm;
    umax = (Gmax/(flowarea*rho))*(TPitch/(TPitch-BattD));                   %peak air speed within pack
    [Re,Pr,Gr,k,Cpa] = Variablefinder('air',filmT1,airtemp,umax,BattD);     %re-find variables based on speed
end

[Res,Prs,Grs,ks,Cps] = Variablefinder('air',BattT,BattT,umax,BattD);

if GrN/(Re^2) < 1
    if Re < 100
        C1 = 0.9;
        m = 0.4;
        n = 0.36;
    elseif Re < 1000
        C1 = 0.52;
        m = 0.5;
        n = 0.36;
    elseif Re < (2*(10^5))
        C1 = 0.27;
        m = 0.63;
        n = 0.36;
    else
        C1 = 0.033;
        m = 0.8;
        n = 0.4;
    end
C2 = 1;
    switch Nl
        case (1)
            C2 = 0.7;    
        case (2)
            C2 = 0.8;
        case (3)
            C2 = 0.86;
        case (4)
            C2 = 0.9;
        case (5)
            C2 = 0.92;
        case(7)
            C2 = 0.95;
        case(10)
            C2 = 0.97;
        case(13)
            C2 = 0.98;
        case(16)
            C2 = 0.99;
        case(20)
            C2 = 1;
    end

    Nu = C2*C1*(Re^m)*(Pr^n)*((Pr/Prs)^0.25);
    
    h = Nu*k/(BattD);
    R = 1/( (Nt*Nv*Nl*BattD*pi()*BattL) * h );
    
    airout = BattT - (BattT-airtemp)*exp(-1/(Gmax*Cpa*R));        %(h*(Nt*Nl*BattD*pi()*BattL))
    %airout = ( BattT + ((Gmax*Cpa*R) - 1/2)*airtemp ) / ((Gmax*Cpa*R) + 1/2);
    LossA = Gmax*Cpa*(airout-airtemp);
else
    Ra = PrN*GrN;  %calculate the rayleigh number
    Nu = (0.68 + ( (0.387*(Ra^(1/6))) / ((1 + ((0.492/PrN)^(9/16)))^(8/27)) ) )^2;
    %Nu = 0.478*(GrN^0.25);
    
    h = Nu*k/(BattL*Nv);
    R = 1/( (Nt*Nv*Nl*BattD*pi()*BattL) * h );
    LossA = (BattT-((airtemp+BattT)/2))/R;
end

end

== matlab function ThermalModel/Calc block/Pipe2/MATLAB Function ==
  data: airtemp input; waterin input; waterout output; pipelength input; ID input; OD input
function waterout = Pipefcn(airtemp,waterin,pipelength,ID,OD)

L = pipelength;
AveWtemp = waterin;
kpipe = 0.13;
dm = 0.1;
u = (dm/1000)/(pi()*((ID/2)^2));
filmT1 = (waterin + airtemp)/2;
filmT2 = (waterin + airtemp)/2;

for x = 1:3
    [Rew,Prw,Grw,kw,Cpw] = Variablefinder('water',filmT1,AveWtemp,u,ID);
    [Rea,Pra,Gra,ka,Cpa] = Variablefinder('air',filmT2,airtemp,0,OD);
    
    if Rew <= 2300
        Nuw = 3.66;     %value for laminar flow in a pipe with constant surface temp
    else
       Nuw = 0.023*(Rew^(4/5))*(Prw^0.3);   %equation for turbulent flow in a cooling pipe
    end
    
    Raa = Pra*Gra;  %calculate the rayleigh number
    HorNua = (0.6 + ( (0.387*(Raa^(1/6))) / ((1 + ((0.559/Pra)^(9/16)))^(8/27)) ) )^2;
    VertNua = (0.825 + ( (0.387*(Raa^(1/6))) / ((1 + ((0.492/Pra)^(9/16)))^(8/27)) ) )^2;
    Nua = 1*HorNua + 0*VertNua;
    
    h1 = Nuw*kw/ID;
    h2 = Nua*ka/OD;

    R1 = 1/(2*pi()*(ID/2)*L*h1);
    R2 = (log((OD/2)/(ID/2)))/(2*pi()*L*kpipe);
    R3 = 1/(2*pi()*(OD/2)*L*h2);
    Rt = R1 + R2 + R3;
    
    waterout = airtemp - (airtemp-waterin)*exp(-1/(dm*Cpw*Rt));

    AveWtemp = (waterin + waterout)/2;
    AvedQ = dm*Cpw*(waterin - waterout);
    
    dTt = AveWtemp - airtemp;
    dT1 = dTt*(R1/Rt);
    dT3 = dTt*(R3/Rt);
    
    filmT1 = AveWtemp - (dT1/2);
    filmT2 = airtemp + (dT3/2);   
end

end

== matlab function ThermalModel/Calc block/Pipe/MATLAB Function ==
  data: airtemp input; waterin input; waterout output; pipelength input; ID input; OD input
function waterout = Pipefcn(airtemp,waterin,pipelength,ID,OD)

L = pipelength;
AveWtemp = waterin;
kpipe = 0.13;
dm = 0.1;
u = (dm/1000)/(pi()*((ID/2)^2));
filmT1 = (waterin + airtemp)/2;
filmT2 = (waterin + airtemp)/2;

for x = 1:3
    [Rew,Prw,Grw,kw,Cpw] = Variablefinder('water',filmT1,AveWtemp,u,ID);
    [Rea,Pra,Gra,ka,Cpa] = Variablefinder('air',filmT2,airtemp,0,OD);
    
    if Rew <= 2300
        Nuw = 3.66;     %value for laminar flow in a pipe with constant surface temp
    else
       Nuw = 0.023*(Rew^(4/5))*(Prw^0.3);   %equation for turbulent flow in a cooling pipe
    end
    
    Raa = Pra*Gra;  %calculate the rayleigh number
    HorNua = (0.6 + ( (0.387*(Raa^(1/6))) / ((1 + ((0.559/Pra)^(9/16)))^(8/27)) ) )^2;
    VertNua = (0.825 + ( (0.387*(Raa^(1/6))) / ((1 + ((0.492/Pra)^(9/16)))^(8/27)) ) )^2;
    Nua = 1*HorNua + 0*VertNua;
    
    h1 = Nuw*kw/ID;
    h2 = Nua*ka/OD;

    R1 = 1/(2*pi()*(ID/2)*L*h1);
    R2 = (log((OD/2)/(ID/2)))/(2*pi()*L*kpipe);
    R3 = 1/(2*pi()*(OD/2)*L*h2);
    Rt = R1 + R2 + R3;
    
    waterout = airtemp - (airtemp-waterin)*exp(-1/(dm*Cpw*Rt));

    AveWtemp = (waterin + waterout)/2;
    AvedQ = dm*Cpw*(waterin - waterout);
    
    dTt = AveWtemp - airtemp;
    dT1 = dTt*(R1/Rt);
    dT3 = dTt*(R3/Rt);
    
    filmT1 = AveWtemp - (dT1/2);
    filmT2 = airtemp + (dT3/2);   
end

end

== matlab function ThermalModel/MATLAB Function ==
  data: u input; y output
function y = fcn(u)
if u == 1
    y = u;
end
y = u;

== matlab function ThermalModel/Calc block/Radiator/MATLAB Function1 ==
  data: airtemp input; airspeed input; waterin input; waterout output; pipelength input; pipeno input; pipespacing input; finpitch input; PipeDepth input; PipeWidth input
function waterout = Radfcn(airtemp,airspeed,waterin,pipelength,pipeno,pipespacing,finpitch,PipeDepth,PipeWidth)

dmw = 0.1;
u = ((dmw/1000)/(PipeDepth*PipeWidth))/pipeno;

L = pipelength;
Hdw = (4*PipeDepth*PipeWidth)/(2*PipeDepth+2*PipeWidth);

k = 205;

AirflowArea = pipelength*pipespacing*(pipeno-1);
Fins = round(pipelength*finpitch);
AirPerim = (2*pipelength*pipeno)+(2*Fins*pipespacing*(pipeno-1));
Hda = (4*AirflowArea)/AirPerim;

AveWtemp = waterin;
filmT1 = (waterin + airtemp)/2;
filmT2 = (waterin + airtemp)/2;

for x = 1:3
    [Rew,Prw,Grw,kw,Cpw] = Variablefinder('water',filmT1,AveWtemp,u,Hdw);
    [Rea,Pra,Gra,ka,Cpa] = Variablefinder('air',filmT2,airtemp,airspeed,Hda);
    
    if Rew <= 2300
        Nuw = 7.54;     %value for laminar flow in a pipe with constant surface temp
    else
        f = (0.79*log(Rew-1.64) )^(-2);
        Nuw = (f/8*(Rew-1000)*Prw)/(1+(12.7*((f/8)^(1/2))*(Prw^(2/3)-1)) );
        %Nuw = 0.023*(Rew^(4/5))*(Prw^0.3);   %equation for turbulent flow in a cooling pipe
    end
    
    if Rea <= 2300
        Nua = 5.6;     %value for laminar flow in a pipe with constant surface temp
    else
        f = (0.79*log(Rea-1.64) )^(-2);
        Nua = (f/8*(Rea-1000)*Pra)/(1+(12.7*((f/8)^(1/2))*(Pra^(2/3)-1)) );
        %Nua = 0.023*(Rea^(4/5))*(Pra^0.3);   %equation for turbulent flow in a 
    end
    
%     if Rea <= (5*10^5)
%         Nua = 0.664*(Rea^(1/2))*(Pra^(1/3));
%     else
%         Nua = ((0.037*(Rea^(4/5)))-871)*(Pra^(1/3));
%     end
    
    h1 = Nuw*kw/Hdw;
    h2 = Nua*ka/Hda;

    Rw = 0.0003/(k*pipelength*PipeDepth);
    
    FinArea = (0.0001*PipeDepth);
    Rf = 0.5*pipespacing/(k*FinArea);
    Rfc = 1/(0.5*PipeDepth*(1/finpitch)*11400);
    Rf = 1/((1/(Rf+Rfc))*Fins);
    
    Rfb = Rfc + 0.0001/(0.5*k*PipeDepth*(1/finpitch));
    Rfb = 1/((1/(Rfb))*(Fins));

    
    R1 = 1/((2*PipeDepth+2*PipeWidth)*L*h1);
    R2 = ((Rw *0.5*(2*pipelength*pipeno)/AirPerim) +((Rw+Rfb)*0.5*(2*pipelength*pipeno)/AirPerim) + ((Rw+Rf) * (2*Fins*pipespacing*(pipeno-1))/AirPerim)) *2; 
    %R2 = 0.08;
    R3 = 1/(AirPerim*PipeDepth*h2);
    Rt = R1 + R2 + R3;
    
    waterout = airtemp - (airtemp-waterin)*exp(-1/(dmw*Cpw*Rt/pipeno));

    AveWtemp = (waterin + waterout)/2;
    AvedQ = dmw*Cpw*(waterin - waterout);
    
    
    dTt = AveWtemp - airtemp;
    dT1 = dTt*(R1/Rt);
    dT3 = dTt*(R3/Rt);
    
    filmT1 = AveWtemp - (dT1/2);
    filmT2 = airtemp + (dT3/2);   
end

end

== matlab function ThermalModel/Calc block/Inverter/MATLAB Function ==
  data: airtemp input; waterin input; CaseTb input; CaseTw input; waterout output; pipelength input; ID input; CaseL input; CaseH input; CaseD input; LossW output; LossA output
function [waterout,LossW,LossA] = Invfcn(airtemp,waterin,CaseTb,CaseTw,pipelength,ID,CaseL,CaseH,CaseD)

CaseTb = CaseTb - 273.15;
CaseTw = CaseTw - 273.15;
u = (0.0001)/(pi()*((ID/2)^2));
dmw = 0.0001*1000;
L = pipelength;
AveWtemp = waterin;
filmT1 = (waterin + CaseTb)/2;
filmT2 = (CaseTw + airtemp)/2;

[Rew,Prw,Grw,kw,Cpw] = Variablefinder('water',filmT1,AveWtemp,u,ID);
[Rea,Pra,Gra,ka,Cpa] = Variablefinder('air',filmT2,airtemp,0,CaseH);

if Rew <= 2300
    Nuw = 3.66;     %value for laminar flow in a pipe with constant surface temp
elseif Rew<= 10000
    f = (0.79*log(Rew-1.64) )^(-2);
    Nuw = (f/8*(Rew-1000)*Prw)/(1+(12.7*((f/8)^(1/2))*(Prw^(2/3)-1)) );
else
    Nuw = 0.023*(Rew^(4/5))*(Prw^0.3);   %equation for turbulent flow in a cooling pipe
end

Raa = Pra*Gra;  %calculate the rayleigh number
Nua = (0.825 + ( (0.387*(Raa^(1/6))) / ((1 + ((0.492/Pra)^(9/16)))^(8/27)) ) )^2;

h1 = Nuw*kw/(ID);
h2 = Nua*ka/CaseH;

R1 = 1/(2*pi()*(ID/2)*L*h1);

R2 = 1/(((2*CaseL*CaseH)+(2*CaseH*CaseD))*h2);

waterout = CaseTb - (CaseTb-waterin)*exp(-1/(dmw*Cpw*R1));

LossW = dmw*Cpw*(waterout - waterin);

LossA = (CaseTw-airtemp)/R2;

end
